simulink model "SprungModule"  (Simulink 7.7)
settings: Solver=ode45  StartTime=0.0  StopTime=750  MaxStep=1  RelTol=1e-3
libraries: simulink x1, aerolibatmos2 x1
settings Model: Creator=andreas  LastModifiedBy=andreas

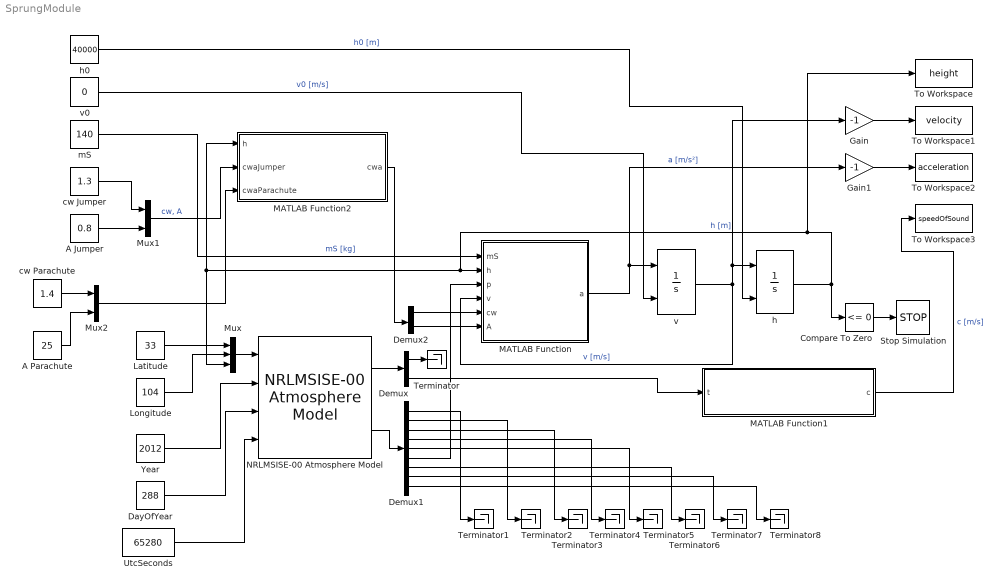
== system SprungModule ==
  A Jumper : Constant  Value=0.8
  A Parachute : Constant  Value=25
  Compare To Zero : simulink/Logic and Bit Operations/Compare To Zero  SystemSampleTime=-1  relop=<=  LogicOutDataTypeMode=boolean
  DayOfYear : Constant  Value=288
  Demux : Demux  Outputs=2
  Demux1 : Demux  Outputs=9
  Demux2 : Demux  Outputs=2
  Gain : Gain  Gain=-1
  Gain1 : Gain  Gain=-1
  Latitude : Constant  Value=33
  Longitude : Constant  Value=104
  MATLAB Function : Stateflow chart  TreatAsAtomicUnit=on
  MATLAB Function1 : Stateflow chart  TreatAsAtomicUnit=on
  MATLAB Function2 : Stateflow chart  TreatAsAtomicUnit=on
  Mux : Mux  Inputs=3
  Mux1 : Mux  Inputs=2
  Mux2 : Mux  Inputs=2
  NRLMSISE-00 Atmosphere Model : aerolibatmos2/NRLMSISE-00 Atmosphere Model  SystemSampleTime=-1  units=Metric (MKS)  lst_input=off  flux_ap_input=off  flags_input=Internal  flags=ones(1,23)  oxygen_in=off  action=Warning
  Stop Simulation : Stop
  Terminator{,1..8} (9 alike) : Terminator
  To Workspace : ToWorkspace  VariableName=height  SampleTime=-1  SaveFormat=Array
  To Workspace1 : ToWorkspace  VariableName=velocity  SampleTime=-1  SaveFormat=Array
  To Workspace2 : ToWorkspace  VariableName=acceleration  SampleTime=-1  SaveFormat=Array
  To Workspace3 : ToWorkspace  VariableName=speedOfSound  SampleTime=-1  SaveFormat=Array
  UtcSeconds : Constant  Value=65280
  Year : Constant  Value=2012
  cw Jumper : Constant  Value=1.3
  cw Parachute : Constant  Value=1.4
  h : Integrator  InitialConditionSource=external
  h0 : Constant  Value=40000
  mS : Constant  Value=140
  v : Integrator  InitialConditionSource=external
  v0 : Constant  Value=0
  wires:
  Latitude/1 -> Mux/1
  Longitude/1 -> Mux/2
  Mux/1 -> NRLMSISE-00 Atmosphere Model/1
  Year/1 -> NRLMSISE-00 Atmosphere Model/2
  DayOfYear/1 -> NRLMSISE-00 Atmosphere Model/3
  UtcSeconds/1 -> NRLMSISE-00 Atmosphere Model/4
  h/1 -> Compare To Zero/1, MATLAB Function/2(h), Mux/3, MATLAB Function2/1(h), To Workspace/1  "h [m]"
  NRLMSISE-00 Atmosphere Model/2 -> Demux1/1
  NRLMSISE-00 Atmosphere Model/1 -> Demux/1
  MATLAB Function/1(a) -> v/1, Gain1/1  "a [m/s²]"
  Demux1/6 -> MATLAB Function/3(p)
  v/1 -> MATLAB Function/4(v), h/1, Gain/1  "v [m/s]"
  Compare To Zero/1 -> Stop Simulation/1
  cw Jumper/1 -> Mux1/1
  A Jumper/1 -> Mux1/2
  Demux2/1 -> MATLAB Function/5(cw)
  Demux2/2 -> MATLAB Function/6(A)
  v0/1 -> v/2  "v0 [m/s]"
  mS/1 -> MATLAB Function/1(mS)  "mS [kg]"
  Demux/1 -> Terminator/1
  Demux/2 -> MATLAB Function1/1(t)
  Demux1/1 -> Terminator1/1
  Demux1/2 -> Terminator2/1
  Demux1/3 -> Terminator3/1
  Demux1/4 -> Terminator4/1
  Demux1/5 -> Terminator5/1
  Demux1/7 -> Terminator6/1
  Demux1/8 -> Terminator7/1
  Demux1/9 -> Terminator8/1
  Gain/1 -> To Workspace1/1
  Gain1/1 -> To Workspace2/1
  h0/1 -> h/2  "h0 [m]"
  MATLAB Function1/1(c) -> To Workspace3/1  "c [m/s]"
  cw Parachute/1 -> Mux2/1
  A Parachute/1 -> Mux2/2
  Mux2/1 -> MATLAB Function2/3(cwaParachute)
  Mux1/1 -> MATLAB Function2/2(cwaJumper)  "cw, A"
  MATLAB Function2/1(cwa) -> Demux2/1

== matlab function MATLAB Function ==
  data: mS input double; a output double; h input double; p input double; v input double; cw input double; A input double
function a = beschleunigung(mS, h, p, v, cw, A)

% Erdmasse
mE=5.9736*10^24;
% Erdradius
rE=6378137;
% Gravitationskonstante
G=66.7384*10^-12;

a=(p/2*v^2*cw*A - (G*(mS*mE)/(rE+h)^2))/mS;

== matlab function MATLAB Function1 ==
  data: t input double; c output double
function c = schallgeschwindigkeit(t)
c = 331.3*sqrt(1 + (t-273.15)/273.15);

== matlab function MATLAB Function2 ==
  data: h input double; cwa output double; cwaJumper input double; cwaParachute input double
function cwa = triggerParachute(h, cwaJumper, cwaParachute)
%#codegen

triggerHeight=1500;


if h>triggerHeight
    cwa=cwaJumper;
else
    cwa=cwaParachute;
end
